simulink library "Springs_Axle3_Linear"  (R2026a)
settings: Solver=VariableStepAuto
undefined symbols (not defined in the file): Spring
libraries: fl_lib x6, Spring_Linear x6
Description:
  | Component of Simscape Vehicle Templates Library
  | 
  | Copyright 2018-2026 The MathWorks, Inc.
settings Model: Creator=smiller  LastModifiedBy=smiller

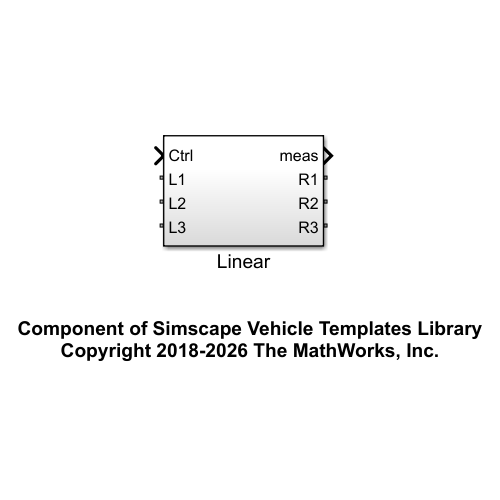
[thumbnail: Simulink's stored preview of the top-level diagram]
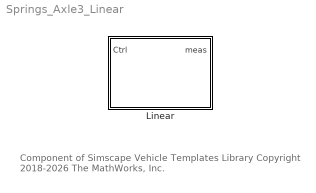
== system Springs_Axle3_Linear ==
  note: Component of Simscape Vehicle Templates Library
      | Copyright 2018-2026 The MathWorks, Inc.
  Linear : Subsystem  VariantControl=Linear

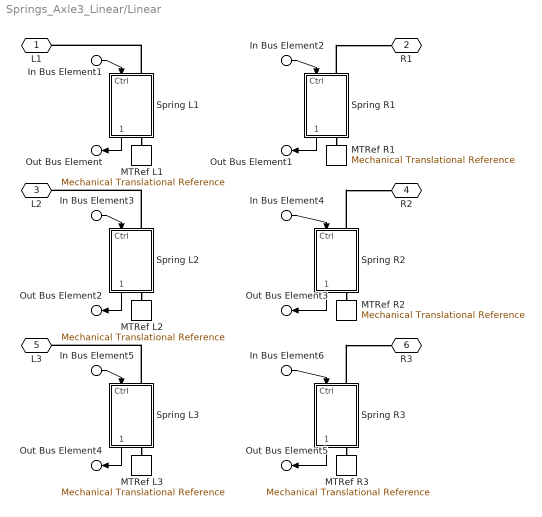
== system Springs_Axle3_Linear/Linear ==
  In Bus Element1 : Inport  PortName=Ctrl  Element=L1
  In Bus Element2 : Inport  PortName=Ctrl  Element=R1
  In Bus Element3 : Inport  PortName=Ctrl  Element=L2
  In Bus Element4 : Inport  PortName=Ctrl  Element=R2
  In Bus Element5 : Inport  PortName=Ctrl  Element=L3
  In Bus Element6 : Inport  PortName=Ctrl  Element=R3
  MTRef L1 : fl_lib/Mechanical/Translational Elements/Mechanical Translational Reference
  MTRef L2 : fl_lib/Mechanical/Translational Elements/Mechanical Translational Reference
  MTRef L3 : fl_lib/Mechanical/Translational Elements/Mechanical Translational Reference
  MTRef R1 : fl_lib/Mechanical/Translational Elements/Mechanical Translational Reference
  MTRef R2 : fl_lib/Mechanical/Translational Elements/Mechanical Translational Reference
  MTRef R3 : fl_lib/Mechanical/Translational Elements/Mechanical Translational Reference
  Spring L1 : Subsystem  mask{Spring=Spring.Axle1}
      mask prompts: Spring "Spring Parameters"
  Spring L2 : Subsystem  mask{Spring=Spring.Axle2}
      mask prompts: Spring "Spring Parameters"
  Spring L3 : Subsystem  mask{Spring=Spring.Axle2}
      mask prompts: Spring "Spring Parameters"
  Spring R1 : Subsystem  mask{Spring=Spring.Axle1}
      mask prompts: Spring "Spring Parameters"
  Spring R2 : Subsystem  mask{Spring=Spring.Axle2}
      mask prompts: Spring "Spring Parameters"
  Spring R3 : Subsystem  mask{Spring=Spring.Axle2}
      mask prompts: Spring "Spring Parameters"
  L1 : PMIOPort  Side=Left
  R1 : PMIOPort  Port=2  Side=Right
  L2 : PMIOPort  Port=3  Side=Left
  R2 : PMIOPort  Port=4  Side=Right
  L3 : PMIOPort  Port=5  Side=Left
  R3 : PMIOPort  Port=6  Side=Right
  Out Bus Element : Outport  VectorParamsAs1DForOutWhenUnconnected=off  PortName=meas  Element=L1
  Out Bus Element1 : Outport  VectorParamsAs1DForOutWhenUnconnected=off  PortName=meas  Element=R1
  Out Bus Element2 : Outport  VectorParamsAs1DForOutWhenUnconnected=off  PortName=meas  Element=L2
  Out Bus Element3 : Outport  VectorParamsAs1DForOutWhenUnconnected=off  PortName=meas  Element=R2
  Out Bus Element4 : Outport  VectorParamsAs1DForOutWhenUnconnected=off  PortName=meas  Element=L3
  Out Bus Element5 : Outport  VectorParamsAs1DForOutWhenUnconnected=off  PortName=meas  Element=R3
  wires:
  In Bus Element1/1 -> Spring L1/1(Ctrl)
  Spring L1/1(meas) -> Out Bus Element/1
  In Bus Element2/1 -> Spring R1/1(Ctrl)
  Spring R1/1(meas) -> Out Bus Element1/1
  In Bus Element3/1 -> Spring L2/1(Ctrl)
  Spring L2/1(meas) -> Out Bus Element2/1
  In Bus Element4/1 -> Spring R2/1(Ctrl)
  Spring R2/1(meas) -> Out Bus Element3/1
  Spring R3/1(meas) -> Out Bus Element5/1
  In Bus Element6/1 -> Spring R3/1(Ctrl)
  Spring L3/1(meas) -> Out Bus Element4/1
  In Bus Element5/1 -> Spring L3/1(Ctrl)
  connections:
  Spring R1/LConn1 -- R1/RConn1
  Spring R1/RConn1 -- MTRef R1/LConn1
  Spring R2/LConn1 -- R2/RConn1
  Spring R2/RConn1 -- MTRef R2/LConn1
  Spring L2/LConn1 -- L2/RConn1
  Spring L2/RConn1 -- MTRef L2/LConn1
  Spring L1/LConn1 -- L1/RConn1
  Spring L1/RConn1 -- MTRef L1/LConn1
  Spring L3/RConn1 -- MTRef L3/LConn1
  Spring L3/LConn1 -- L3/RConn1
  Spring R3/RConn1 -- MTRef R3/LConn1
  Spring R3/LConn1 -- R3/RConn1

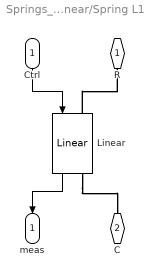
== system Springs_Axle3_Linear/Linear/Spring L1 ==
  Ctrl : Inport
  Linear : Spring_Linear/Linear  VariantControl=Linear  spr_def0=Spring.xPreload.Value  spr_frc0=Spring.fPreload.Value  spr_k=Spring.K.Value  spr_hp_top=Spring.sTop.Value  spr_hp_bot=Spring.sBottom.Value
  R : PMIOPort  Side=Left
  C : PMIOPort  Port=2  Side=Right
  meas : Outport  VectorParamsAs1DForOutWhenUnconnected=off
  wires:
  Linear/1 -> meas/1
  Ctrl/1 -> Linear/1
  connections:
  Linear/LConn1 -- R/RConn1
  Linear/RConn1 -- C/RConn1

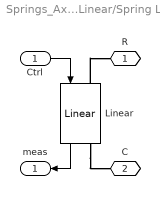
== system Springs_Axle3_Linear/Linear/Spring L2 ==
  Ctrl : Inport
  Linear : Spring_Linear/Linear  VariantControl=Linear  spr_def0=Spring.xPreload.Value  spr_frc0=Spring.fPreload.Value  spr_k=Spring.K.Value  spr_hp_top=Spring.sTop.Value  spr_hp_bot=Spring.sBottom.Value
  R : PMIOPort  Side=Left
  C : PMIOPort  Port=2  Side=Right
  meas : Outport  VectorParamsAs1DForOutWhenUnconnected=off
  wires:
  Ctrl/1 -> Linear/1
  Linear/1 -> meas/1
  connections:
  Linear/RConn1 -- C/RConn1
  Linear/LConn1 -- R/RConn1

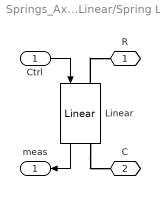
== system Springs_Axle3_Linear/Linear/Spring L3 ==
  Ctrl : Inport
  Linear : Spring_Linear/Linear  VariantControl=Linear  spr_def0=Spring.xPreload.Value  spr_frc0=Spring.fPreload.Value  spr_k=Spring.K.Value  spr_hp_top=Spring.sTop.Value  spr_hp_bot=Spring.sBottom.Value
  R : PMIOPort  Side=Left
  C : PMIOPort  Port=2  Side=Right
  meas : Outport  VectorParamsAs1DForOutWhenUnconnected=off
  wires:
  Linear/1 -> meas/1
  Ctrl/1 -> Linear/1
  connections:
  Linear/LConn1 -- R/RConn1
  Linear/RConn1 -- C/RConn1

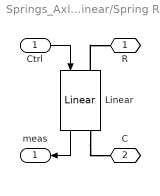
== system Springs_Axle3_Linear/Linear/Spring R1 ==
  Ctrl : Inport
  Linear : Spring_Linear/Linear  VariantControl=Linear  spr_def0=Spring.xPreload.Value  spr_frc0=Spring.fPreload.Value  spr_k=Spring.K.Value  spr_hp_top=Spring.sTop.Value  spr_hp_bot=Spring.sBottom.Value
  R : PMIOPort  Side=Left
  C : PMIOPort  Port=2  Side=Right
  meas : Outport  VectorParamsAs1DForOutWhenUnconnected=off
  wires:
  Ctrl/1 -> Linear/1
  Linear/1 -> meas/1
  connections:
  Linear/RConn1 -- C/RConn1
  Linear/LConn1 -- R/RConn1

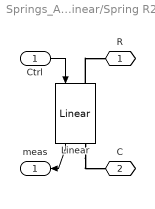
== system Springs_Axle3_Linear/Linear/Spring R2 ==
  Ctrl : Inport
  Linear : Spring_Linear/Linear  VariantControl=Linear  spr_def0=Spring.xPreload.Value  spr_frc0=Spring.fPreload.Value  spr_k=Spring.K.Value  spr_hp_top=Spring.sTop.Value  spr_hp_bot=Spring.sBottom.Value
  R : PMIOPort  Side=Left
  C : PMIOPort  Port=2  Side=Right
  meas : Outport  VectorParamsAs1DForOutWhenUnconnected=off
  wires:
  Linear/1 -> meas/1
  Ctrl/1 -> Linear/1
  connections:
  Linear/LConn1 -- R/RConn1
  Linear/RConn1 -- C/RConn1

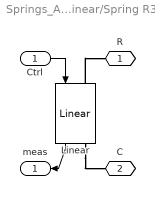
== system Springs_Axle3_Linear/Linear/Spring R3 ==
  Ctrl : Inport
  Linear : Spring_Linear/Linear  VariantControl=Linear  spr_def0=Spring.xPreload.Value  spr_frc0=Spring.fPreload.Value  spr_k=Spring.K.Value  spr_hp_top=Spring.sTop.Value  spr_hp_bot=Spring.sBottom.Value
  R : PMIOPort  Side=Left
  C : PMIOPort  Port=2  Side=Right
  meas : Outport  VectorParamsAs1DForOutWhenUnconnected=off
  wires:
  Ctrl/1 -> Linear/1
  Linear/1 -> meas/1
  connections:
  Linear/RConn1 -- C/RConn1
  Linear/LConn1 -- R/RConn1
